simulink model "CurrPowerLimCalc"  (R2022b)
settings: configuration reference "BMS_Sw_CodeGenConfig" (kept outside this file)
undefined symbols (not defined in the file): HighCellTempLimit, LowCellTempLimit, MaxChrgCurrLim, MaxDchrgCurrLim, MinCellVoltDchrgCurrentLim_BP, MinCellVoltDchrgCurrentLim_Table, Np_Module, OverCellVoltageLimit, UnderCellVoltageLimit
libraries: FaultManagement_lib x6, simulink x5
settings Model: DataDictionary=DD_CurrPowerLimCalc.sldd  EnableAccessToBaseWorkspace=off  ExtModeTrigDuration=5  Creator=cpatel  LastModifiedBy=cpatel
settings ConfigSetRef: SourceName=BMS_Sw_CodeGenConfig

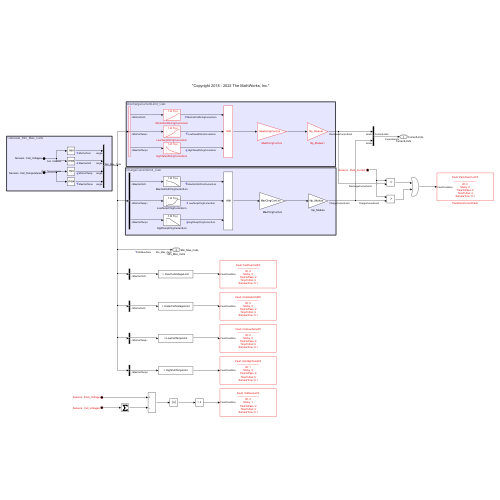
[thumbnail: Simulink's stored preview of the top-level diagram]
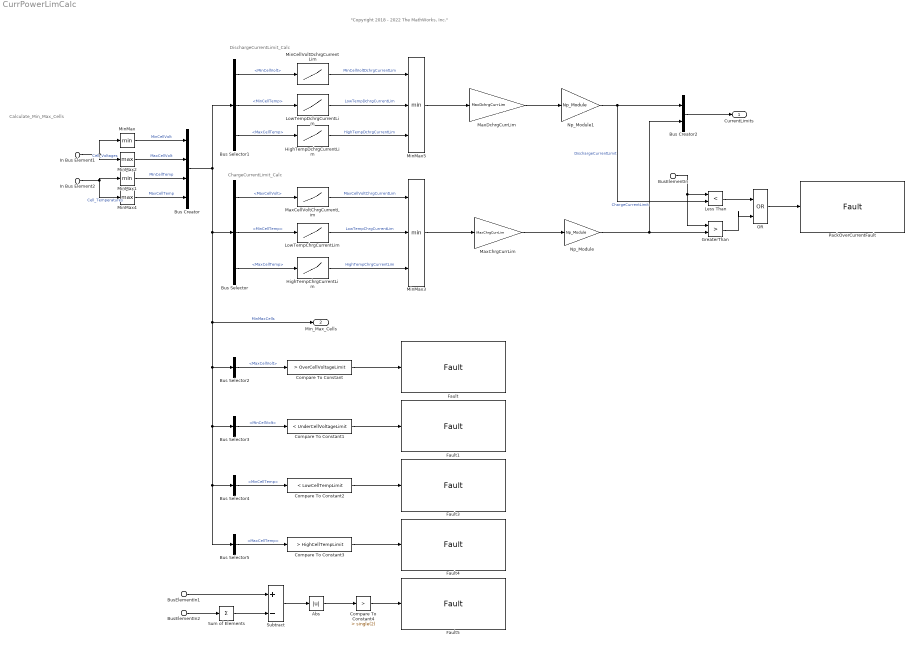
== system CurrPowerLimCalc ==
  note: ChargeCurrentLimit_Calc
  note: Calculate_Min_Max_Cells
  note: "Copyright 2018 - 2022 The MathWorks, Inc."
  note: DischargeCurrentLimit_Calc
  In Bus Element1 : Inport  PortName=Sensors  Element=Cell_Voltages
  BusElementIn2 : Inport  PortName=Sensors  Element=Cell_Voltages
  BusElementIn1 : Inport  PortName=Sensors  Element=Pack_Voltage
  BusElementIn : Inport  PortName=Sensors  Element=Pack_Current
  In Bus Element2 : Inport  PortName=Sensors  Element=Cell_Temperatures
  Abs : Abs  SaturateOnIntegerOverflow=off
  Bus Creator : BusCreator  Inputs=4  OutDataTypeStr=Bus: Min_Max_Cells  NonVirtualBus=on
      settings: InheritFromInputs=off
  Bus Selector : BusSelector  OutputSignals=MaxCellVolt,MinCellTemp,MaxCellTemp
  Bus Selector1 : BusSelector  OutputSignals=MinCellVolt,MinCellTemp,MaxCellTemp
  Bus Selector2 : BusSelector  OutputSignals=MaxCellVolt
  Bus Selector3 : BusSelector  OutputSignals=MinCellVolt
  Bus Selector4 : BusSelector  OutputSignals=MinCellTemp
  Bus Selector5 : BusSelector  OutputSignals=MaxCellTemp
  Bus Creator2 : BusCreator  Inputs=2  OutDataTypeStr=Bus: CurrentLimits  NonVirtualBus=on
  Compare To Constant : simulink/Logic and Bit Operations/Compare To Constant  relop=>  const=OverCellVoltageLimit  OutDataTypeStr=boolean
  Compare To Constant1 : simulink/Logic and Bit Operations/Compare To Constant  relop=<  const=UnderCellVoltageLimit  OutDataTypeStr=boolean
  Compare To Constant2 : simulink/Logic and Bit Operations/Compare To Constant  relop=<  const=LowCellTempLimit  OutDataTypeStr=boolean
  Compare To Constant3 : simulink/Logic and Bit Operations/Compare To Constant  relop=>  const=HighCellTempLimit  OutDataTypeStr=boolean
  Compare To Constant4 : simulink/Logic and Bit Operations/Compare To Constant  relop=>  const=single(2)  OutDataTypeStr=boolean
  Fault : FaultManagement_lib/Fault  FaultName=CellOverVoltFlt  ID=4  Enable=1  Sticky=0  TimeToFail=2  TimeToPass=4  SampleTime=0.1
  Fault1 : FaultManagement_lib/Fault  FaultName=CellUnderVoltFlt  ID=5  Enable=1  Sticky=0  TimeToFail=2  TimeToPass=4  SampleTime=0.1
  Fault3 : FaultManagement_lib/Fault  FaultName=CellLowTempFlt  ID=2  Enable=1  Sticky=0  TimeToFail=4  TimeToPass=6  SampleTime=0.1
  Fault4 : FaultManagement_lib/Fault  FaultName=CellHighTempFlt  ID=1  Enable=1  Sticky=0  TimeToFail=4  TimeToPass=6  SampleTime=0.1
  Fault5 : FaultManagement_lib/Fault  FaultName=VoltSensorFlt  ID=3  Enable=1  Sticky=1  TimeToFail=2  TimeToPass=4  SampleTime=0.1
  GreaterThan : RelationalOperator  Operator=>  OutDataTypeStr=boolean  RndMeth=Simplest  InputSameDT=off
  HighTempChrgCurrentLim : Lookup_n-D  NumberOfTableDimensions=1  BreakpointsForDimension1="single([40  45  50    55 65])"  Table=single([1.0 1.0 0.75 0.5 0])  ExtrapMethod=Clip  InternalRulePriority=Speed  RndMeth=Simplest
  HighTempDchrgCurrentLim : Lookup_n-D  NumberOfTableDimensions=1  BreakpointsForDimension1=single([40, 45, 50, 60])  Table=single([1, 0.5, 0.3, 0])  ExtrapMethod=Clip  InternalRulePriority=Speed  RndMeth=Simplest
  Less Than : RelationalOperator  Operator=<  OutDataTypeStr=boolean  RndMeth=Simplest  InputSameDT=off
  LowTempChrgCurrentLim : Lookup_n-D  NumberOfTableDimensions=1  BreakpointsForDimension1=single([-15 -10 -5.0 0.0 5.0 10 15.0])  Table="single([0.1 0.2  0.3 0.3 0.5 1.0 1.0])"  ExtrapMethod=Clip  InternalRulePriority=Speed  RndMeth=Simplest
  LowTempDchrgCurrentLim : Lookup_n-D  NumberOfTableDimensions=1  BreakpointsForDimension1="single([-10, -5,    0,   5, 10, 15, 20])"  Table="single([0,  0.2, 0.3, 0.5, 0.75, 1, 1])"  ExtrapMethod=Clip  InternalRulePriority=Speed  RndMeth=Simplest
  MaxCellVoltChrgCurrentLim : Lookup_n-D  NumberOfTableDimensions=1  BreakpointsForDimension1=single([4.0 4.10 4.15 4.2])  Table=single([1.0 0.75 0.50 0.2])  ExtrapMethod=Clip  InternalRulePriority=Speed  RndMeth=Simplest
  MaxChrgCurrLim : Gain  Gain=MaxChrgCurrLim
  MaxDchrgCurrLim : Gain  Gain=MaxDchrgCurrLim
  MinCellVoltDchrgCurrentLim : Lookup_n-D  NumberOfTableDimensions=1  DataSpecification=Lookup table object  LookupTableObject=MinCellVoltDchrgCurrentLimTable  BreakpointsForDimension1=MinCellVoltDchrgCurrentLim_BP  Table=MinCellVoltDchrgCurrentLim_Table  ExtrapMethod=Clip  InternalRulePriority=Speed  RndMeth=Simplest
  MinMax : MinMax
  MinMax1 : MinMax
  MinMax2 : MinMax  Function=max
  MinMax3 : MinMax  Inputs=3
  MinMax4 : MinMax  Function=max
  MinMax5 : MinMax  Inputs=3
  Np_Module : Gain  Gain=Np_Module
  Np_Module1 : Gain  Gain=Np_Module
  OR : Logic  Operator=OR  IconShape=distinctive  AllPortsSameDT=off  OutDataTypeStr=boolean
  PackOverCurrentFault : FaultManagement_lib/Fault  FaultName=PackOverCurrFlt  ID=0  Enable=1  Sticky=0  TimeToFail=2  TimeToPass=4  SampleTime=0.1
  Subtract : Sum  Inputs=+-
  Sum of Elements : Sum  Inputs=+
  CurrentLimits : Outport  SignalName=CurrentLimits  OutDataTypeStr=Bus: CurrentLimits  BusOutputAsStruct=on
  Min_Max_Cells : Outport  Port=2  SignalName=Min_Max_Cells  OutDataTypeStr=Bus: Min_Max_Cells  BusOutputAsStruct=on
  wires:
  In Bus Element1/1 -> MinMax/1, MinMax2/1  "Cell_Voltages"
  In Bus Element2/1 -> MinMax4/1, MinMax1/1  "Cell_Temperatures"
  Bus Creator2/1 -> CurrentLimits/1
  Np_Module1/1 -> Bus Creator2/1, Less Than/2  "DischargeCurrentLimit"
  Bus Creator/1 -> Bus Selector/1, Bus Selector5/1, Bus Selector4/1, Bus Selector3/1, Bus Selector2/1, Min_Max_Cells/1, Bus Selector1/1  "MinMaxCells"
  MinMax4/1 -> Bus Creator/4  "MaxCellTemp"
  MinMax1/1 -> Bus Creator/3  "MinCellTemp"
  MinMax/1 -> Bus Creator/1  "MinCellVolt"
  MinMax2/1 -> Bus Creator/2  "MaxCellVolt"
  Np_Module/1 -> Bus Creator2/2, GreaterThan/2  "ChargeCurrentLimit"
  Bus Selector/1 -> MaxCellVoltChrgCurrentLim/1  "<MaxCellVolt>"
  MaxCellVoltChrgCurrentLim/1 -> MinMax3/1  "MaxCellVoltChrgCurrentLim"
  Bus Selector/3 -> HighTempChrgCurrentLim/1  "<MaxCellTemp>"
  Bus Selector/2 -> LowTempChrgCurrentLim/1  "<MinCellTemp>"
  MaxChrgCurrLim/1 -> Np_Module/1
  LowTempChrgCurrentLim/1 -> MinMax3/2  "LowTempChrgCurrentLim"
  HighTempChrgCurrentLim/1 -> MinMax3/3  "HighTempChrgCurrentLim"
  MinMax3/1 -> MaxChrgCurrLim/1
  Bus Selector1/1 -> MinCellVoltDchrgCurrentLim/1  "<MinCellVolt>"
  MinCellVoltDchrgCurrentLim/1 -> MinMax5/1  "MinCellVoltDchrgCurrentLim"
  LowTempDchrgCurrentLim/1 -> MinMax5/2  "LowTempDchrgCurrentLim"
  HighTempDchrgCurrentLim/1 -> MinMax5/3  "HighTempDchrgCurrentLim"
  Bus Selector1/2 -> LowTempDchrgCurrentLim/1  "<MinCellTemp>"
  Bus Selector1/3 -> HighTempDchrgCurrentLim/1  "<MaxCellTemp>"
  MaxDchrgCurrLim/1 -> Np_Module1/1
  MinMax5/1 -> MaxDchrgCurrLim/1
  Bus Selector2/1 -> Compare To Constant/1  "<MaxCellVolt>"
  Compare To Constant1/1 -> Fault1/1
  Compare To Constant/1 -> Fault/1
  Bus Selector3/1 -> Compare To Constant1/1  "<MinCellVolt>"
  BusElementIn/1 -> GreaterThan/1, Less Than/1
  Less Than/1 -> OR/1
  GreaterThan/1 -> OR/2
  OR/1 -> PackOverCurrentFault/1
  Bus Selector4/1 -> Compare To Constant2/1  "<MinCellTemp>"
  Bus Selector5/1 -> Compare To Constant3/1  "<MaxCellTemp>"
  Compare To Constant2/1 -> Fault3/1
  Compare To Constant3/1 -> Fault4/1
  BusElementIn2/1 -> Sum of Elements/1
  Sum of Elements/1 -> Subtract/2
  BusElementIn1/1 -> Subtract/1
  Subtract/1 -> Abs/1
  Abs/1 -> Compare To Constant4/1
  Compare To Constant4/1 -> Fault5/1
